simulink model "punto3"  (Simulink 5.0)
settings: Solver=ode45  StartTime=0.0  StopTime=100.0  RelTol=1e-3
settings Model: LastModifiedBy=Juan

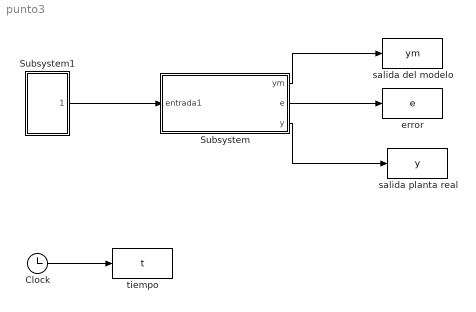
== system punto3 ==
  Clock : Clock
      settings: Decimation=10
  Subsystem : Subsystem  mask{am1=1, am2=1, a1=1, a2=1, kp=1, km=1, g=0.1, titainicial=0}
      mask prompts: am1 "a1 del modelo (am1)"; am2 "a2 del modelo (am2)"; a1 "a1 de la planta real (a1)"; a2 "a2 de la planta real (a2)"; kp "ganancia de la planta real (kp)"; km "ganancia del modelo (km)"; g "gama"; titainicial "valor inicial de tita"
      mask Display: disp('Sistema')
  Subsystem1 : Subsystem  mask{w=3.5}
      mask prompts: w "Amplitud"
  error : ToWorkspace  VariableName=e  SampleTime=-1  SaveFormat=Array
  salida del modelo : ToWorkspace  VariableName=ym  SampleTime=-1  SaveFormat=Array
  salida planta real : ToWorkspace  VariableName=y  SampleTime=-1  SaveFormat=Array
  tiempo : ToWorkspace  VariableName=t  SampleTime=-1  SaveFormat=Array
  wires:
  Clock/1 -> tiempo/1
  Subsystem/1(ym) -> salida del modelo/1
  Subsystem1/1(Entrada) -> Subsystem/1(entrada1)
  Subsystem/2(e) -> error/1
  Subsystem/3(y) -> salida planta real/1

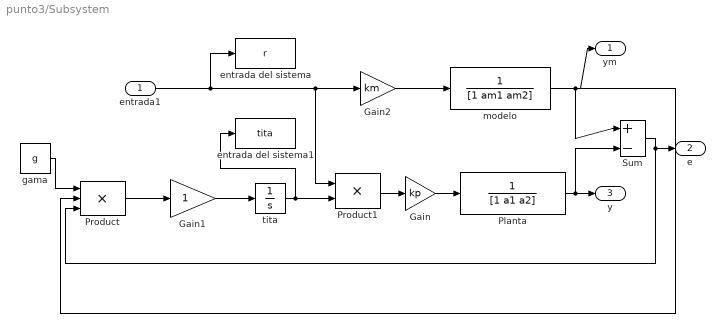
== system punto3/Subsystem ==
  entrada1 : Inport
  Gain : Gain  Gain=kp  SaturateOnIntegerOverflow=on
  Gain1 : Gain  SaturateOnIntegerOverflow=on
  Gain2 : Gain  Gain=km  SaturateOnIntegerOverflow=on
  Planta : TransferFcn  Numerator=1  Denominator=[1 a1 a2]
  Product : Product  Inputs=3  SaturateOnIntegerOverflow=on
  Product1 : Product  SaturateOnIntegerOverflow=on
  Sum : Sum  Inputs=|+-  SaturateOnIntegerOverflow=on
  entrada del sistema : ToWorkspace  VariableName=r  SampleTime=-1  SaveFormat=Array
  entrada del sistema1 : ToWorkspace  VariableName=tita  SampleTime=-1  SaveFormat=Array
  gama : Constant  Value=g
  modelo : TransferFcn  Numerator=1  Denominator=[1 am1 am2]
  tita : Integrator  InitialCondition=titainicial
  ym : Outport
  e : Outport  Port=2
  y : Outport  Port=3
  wires:
  Product/1 -> Gain1/1
  modelo/1 -> Sum/1, Product/2, ym/1
  Planta/1 -> Sum/2, y/1
  Product1/1 -> Gain/1
  tita/1 -> Product1/2, entrada del sistema1/1
  Gain1/1 -> tita/1
  Sum/1 -> Product/3, e/1
  gama/1 -> Product/1
  Gain2/1 -> modelo/1
  Gain/1 -> Planta/1
  entrada1/1 -> entrada del sistema/1, Product1/1, Gain2/1

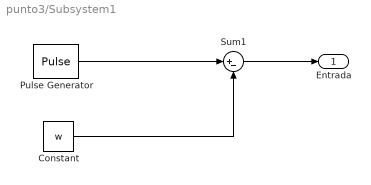
== system punto3/Subsystem1 ==
  Constant : Constant  Value=w
  Pulse Generator : DiscretePulseGenerator  PulseType=Time based  Amplitude=w*2  Period=40  PulseWidth=50
  Sum1 : Sum  Inputs=|+-  SaturateOnIntegerOverflow=on
  Entrada : Outport
  wires:
  Constant/1 -> Sum1/2
  Pulse Generator/1 -> Sum1/1
  Sum1/1 -> Entrada/1
